simulink model "cont_desl"  (R2020a)
settings: Solver=VariableStepAuto  StartTime=0.0  StopTime=15  RelTol=1e-3
settings Model: Creator=Mateus Gilbert  LastModifiedBy=Mateus Gilbert

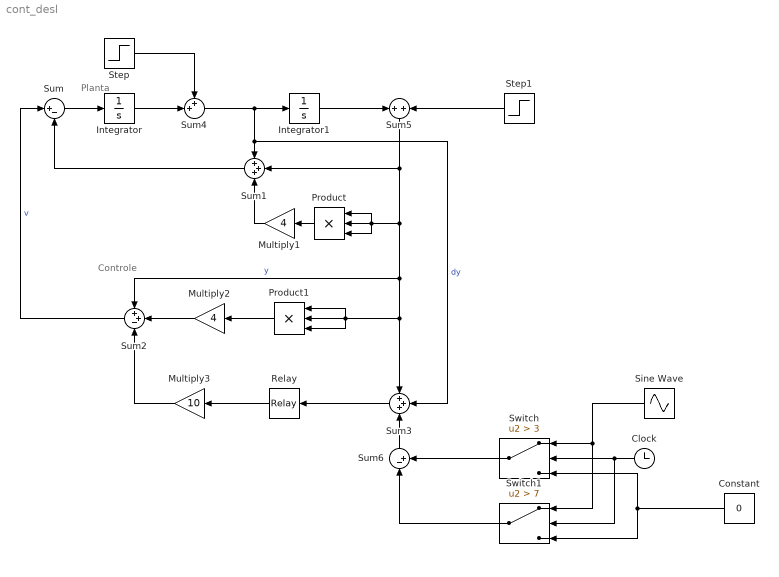
== system cont_desl ==
  note: Planta
  note: Controle
  Clock : Clock
      settings: Decimation=5000
  Constant : Constant  Value=0
  Integrator : Integrator
  Integrator1 : Integrator
  Multiply1 : Gain  Gain=4
  Multiply2 : Gain  Gain=4
  Multiply3 : Gain  Gain=10
  Product : Product  Inputs=3
  Product1 : Product  Inputs=3
  Relay : Relay  OnSwitchValue=1e-5  OffSwitchValue=-1e-5  OffOutputValue=-1
  Sine Wave : Sin  Amplitude=5  Frequency=16*pi  SampleTime=0
  Step : Step  Time=0  After=3  SampleTime=1e-5
  Step1 : Step  Time=0  After=6  SampleTime=1e-5
  Sum : Sum  Inputs=|+-
  Sum1 : Sum  Inputs=+++
  Sum2 : Sum  Inputs=++-
  Sum3 : Sum  Inputs=+++
  Sum4 : Sum  Inputs=++|
  Sum5 : Sum  Inputs=+|+
  Sum6 : Sum  Inputs=|-+
  Switch : Switch  Criteria=u2 > Threshold  Threshold=3
  Switch1 : Switch  Criteria=u2 > Threshold  Threshold=7
  wires:
  Sum/1 -> Integrator/1
  Sum1/1 -> Sum/2
  Product1/1 -> Multiply2/1
  Relay/1 -> Multiply3/1
  Sum3/1 -> Relay/1
  Sum4/1 -> Sum3/2, Sum1/1, Integrator1/1  "dy"
  Integrator/1 -> Sum4/2
  Integrator1/1 -> Sum5/1
  Sum5/1 -> Sum1/2, Product/1, Product/3, Product/2, Sum2/1, Product1/3, Product1/1, Product1/2, Sum3/1  "y"
  Product/1 -> Multiply1/1
  Multiply1/1 -> Sum1/3
  Multiply2/1 -> Sum2/2
  Step/1 -> Sum4/1
  Step1/1 -> Sum5/2
  Sum2/1 -> Sum/1  "v"
  Multiply3/1 -> Sum2/3
  Switch/1 -> Sum6/2
  Sine Wave/1 -> Switch1/1, Switch/1
  Constant/1 -> Switch1/3, Switch/3
  Clock/1 -> Switch/2, Switch1/2
  Sum6/1 -> Sum3/3
  Switch1/1 -> Sum6/1
